simulink model "control_pos_3dof_conMI"  (R2023b)
settings: Solver=ode45  StartTime=0.0  StopTime=tsim  FixedStep=tstep  MaxStep=tstep  RelTol=1e-3
undefined symbols (not defined in the file): a0, a1, MI_Contr1, MI_Contr2, MI_Contr3, MI_motor1, MI_motor2, MI_motor3, robot_params, sigbuilder_block, t_qeq_init, t_tr_init, tau_L
(part 1 of 4)
settings Model: Creator=HP  LastModifiedBy=HP

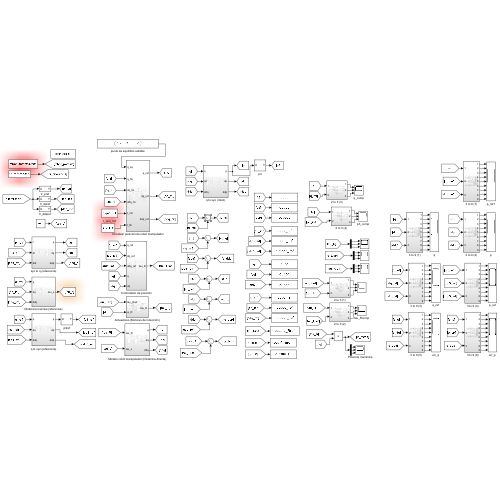
[thumbnail: Simulink's stored preview of the top-level diagram]
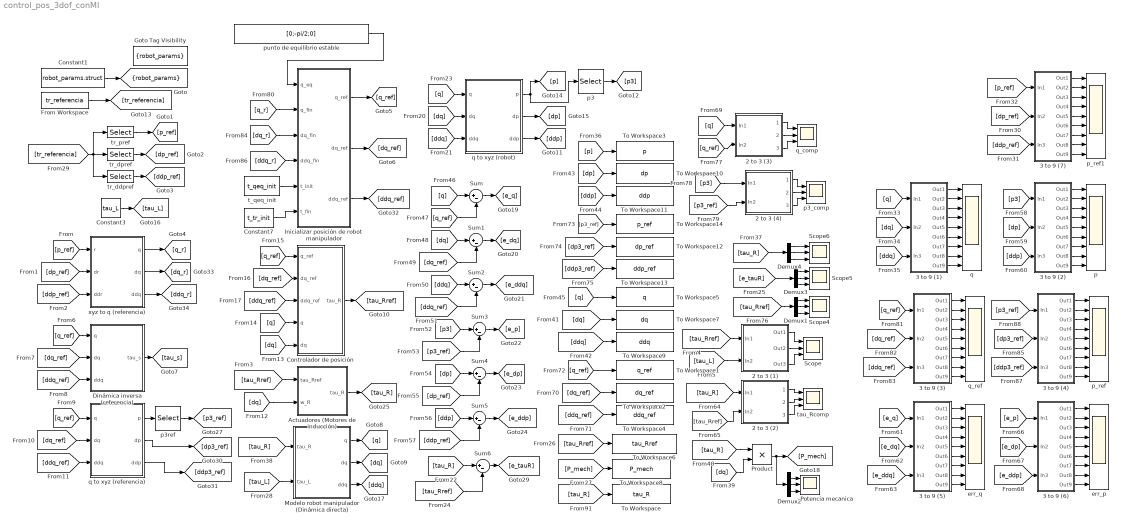
== system control_pos_3dof_conMI ==
  2 to 3 (1) : Subsystem
  2 to 3 (2) : Subsystem
  2 to 3 (3) : Subsystem
  2 to 3 (4) : Subsystem
  3 to 9 (1) : Subsystem
  3 to 9 (2) : Subsystem
  3 to 9 (3) : Subsystem
  3 to 9 (4) : Subsystem
  3 to 9 (5) : Subsystem
  3 to 9 (6) : Subsystem
  3 to 9 (7) : Subsystem
  Actuadores (Motores de inducción) : Subsystem
  Constant1 : Constant  Value=robot_params.struct  OutDataTypeStr=Bus: robot_params_bus
  Constant3 : Constant  Value=tau_L
  Constant7 : Constant  Value=t_tr_init
  Controlador de posición : Subsystem
  Demux{1..4} (4 alike) : Demux  Outputs=3
  Dinámica inversa (referencia) : Subsystem
  From Workspace : FromWorkspace  VariableName=tr_referencia
  Goto Tag Visibility : GotoTagVisibility  GotoTag=robot_params
  Inicializar posición de robot manipulador : Subsystem
  Modelo robot manipulador (Dinámica directa) : Subsystem
  Potencia mecanica : Scope  NumInputPorts=3
  Product : Product
  Scope{,4..6} (4 alike) : Scope  NumInputPorts=3
  Sum{,1..6} (7 alike) : Sum  Inputs=|+-
  To Workspace : ToWorkspace  VariableName=tau_R  SaveFormat=Timeseries  SampleTime=-1
  To Workspace1 : ToWorkspace  VariableName=q_ref  SaveFormat=Timeseries  SampleTime=-1
  To Workspace10 : ToWorkspace  VariableName=dp  SaveFormat=Timeseries  SampleTime=-1
  To Workspace11 : ToWorkspace  VariableName=ddp  SaveFormat=Timeseries  SampleTime=-1
  To Workspace12 : ToWorkspace  VariableName=dp_ref  SaveFormat=Timeseries  SampleTime=-1
  To Workspace13 : ToWorkspace  VariableName=ddp_ref  SaveFormat=Timeseries  SampleTime=-1
  To Workspace14 : ToWorkspace  VariableName=p_ref  SaveFormat=Timeseries  SampleTime=-1
  To Workspace2 : ToWorkspace  VariableName=dq_ref  SaveFormat=Timeseries  SampleTime=-1
  To Workspace3 : ToWorkspace  VariableName=p  SaveFormat=Timeseries  SampleTime=-1
  To Workspace4 : ToWorkspace  VariableName=ddq_ref  SaveFormat=Timeseries  SampleTime=-1
  To Workspace5 : ToWorkspace  VariableName=q  SaveFormat=Timeseries  SampleTime=-1
  To Workspace6 : ToWorkspace  VariableName=tau_Rref  SaveFormat=Timeseries  SampleTime=-1
  To Workspace7 : ToWorkspace  VariableName=dq  SaveFormat=Timeseries  SampleTime=-1
  To Workspace8 : ToWorkspace  VariableName=P_mech  SaveFormat=Timeseries  SampleTime=-1
  To Workspace9 : ToWorkspace  VariableName=ddq  SaveFormat=Timeseries  SampleTime=-1
  err_p : Scope  NumInputPorts=9
  err_q : Scope  NumInputPorts=9
  p : Scope  NumInputPorts=9
  p3 : Selector  NumberOfDimensions=2  InputPortWidth=3  IndexOptions=Index vector (dialog),Index vector (dialog)  Indices=[1:3],3  OutputSizes=1,1
  p3_comp : Scope  NumInputPorts=3
  p3ref : Selector  NumberOfDimensions=2  InputPortWidth=3  IndexOptions=Index vector (dialog),Index vector (dialog)  Indices=[1:3],3  OutputSizes=1,1
  p_ref : Scope  NumInputPorts=9
  p_ref1 : Scope  NumInputPorts=9
  punto de equilibrio estable : Constant  Value=[0;-pi/2;0]
  q : Scope  NumInputPorts=9
  q to xyz (referencia) : Subsystem
  q to xyz (robot) : Subsystem
  q_comp : Scope  NumInputPorts=3
  q_ref : Scope  NumInputPorts=9
  t_qeq_init : Constant  Value=t_qeq_init
  tau_Rcomp : Scope  NumInputPorts=3
  tr_ddpref : Selector  NumberOfDimensions=2  InputPortWidth=3  IndexOptions=Index vector (dialog),Index vector (dialog)  Indices=[7:9],1  OutputSizes=1,1
  tr_dpref : Selector  NumberOfDimensions=2  InputPortWidth=3  IndexOptions=Index vector (dialog),Index vector (dialog)  Indices=[4:6],1  OutputSizes=1,1
  tr_pref : Selector  NumberOfDimensions=2  InputPortWidth=3  IndexOptions=Index vector (dialog),Index vector (dialog)  Indices=[1:3],1  OutputSizes=1,1
  xyz to q (referencia) : Subsystem
  tag scope: robot_params=scoped
  wires:
  From Workspace/1 -> [tr_referencia]
  Constant1/1 -> [robot_params]
  p3/1 -> [p3]
  q to xyz (robot)/2(dp) -> [dp]
  q to xyz (robot)/1(p) -> p3/1, [p]
  [q] -> q to xyz (robot)/1(q)
  [dq] -> q to xyz (robot)/2(dq)
  2 to 3 (1)/2(Out2) -> Scope/2
  [tau_L] -> Modelo robot manipulador (Dinámica directa)/2(tau_L)
  2 to 3 (1)/1(Out1) -> Scope/1
  [tau_R] -> Modelo robot manipulador (Dinámica directa)/1(tau_R)
  [ddq] -> q to xyz (robot)/3(ddq)
  q to xyz (robot)/3(ddp) -> [ddp]
  Constant3/1 -> [tau_L]
  2 to 3 (1)/3(Out3) -> Scope/3
  [tau_R] -> Product/1
  [dq] -> Product/2
  [ddp] -> To Workspace11/1
  Product/1 -> Demux2/1, [P_mech]
  Demux2/3 -> Potencia mecanica/3
  [P_mech] -> To Workspace8/1
  [dq] -> To Workspace7/1
  [q] -> To Workspace5/1
  [tau_Rref] -> To Workspace6/1
  [dp] -> To Workspace10/1
  [p] -> To Workspace3/1
  [ddq] -> To Workspace9/1
  Demux2/2 -> Potencia mecanica/2
  Demux2/1 -> Potencia mecanica/1
  [q] -> Sum/1
  [q_ref] -> Sum/2
  Sum/1 -> [e_q]
  [dq_ref] -> Sum1/2
  Sum1/1 -> [e_dq]
  [dq] -> Sum1/1
  [ddq_ref] -> Sum2/2
  Sum2/1 -> [e_ddq]
  [ddq] -> Sum2/1
  [p3_ref] -> Sum3/2
  Sum4/1 -> [e_dp]
  Sum5/1 -> [e_ddp]
  [ddp_ref] -> Sum5/2
  [dp_ref] -> Sum4/2
  Sum3/1 -> [e_p]
  [p3] -> Sum3/1
  [ddp] -> Sum5/1
  [dp] -> Sum4/1
  p3ref/1 -> [p3_ref]
  [tau_R] -> 2 to 3 (2)/1(In1)
  [tau_Rref] -> 2 to 3 (2)/2(In2)
  2 to 3 (2)/1(1) -> tau_Rcomp/1
  2 to 3 (2)/2(2) -> tau_Rcomp/2
  2 to 3 (2)/3(3) -> tau_Rcomp/3
  [dq_ref] -> To Workspace2/1
  [ddq_ref] -> To Workspace4/1
  [q_ref] -> To Workspace1/1
  [p3_ref] -> To Workspace14/1
  [dp3_ref] -> To Workspace12/1
  [ddp3_ref] -> To Workspace13/1
  [p_ref] -> xyz to q (referencia)/1(r)
  [dp_ref] -> xyz to q (referencia)/2(dr)
  [ddp_ref] -> xyz to q (referencia)/3(ddr)
  [q_ref] -> Dinámica inversa (referencia)/1(q)
  [dq_ref] -> Dinámica inversa (referencia)/2(dq)
  [ddq_ref] -> Dinámica inversa (referencia)/3(ddq)
  Dinámica inversa (referencia)/1(tau_s) -> [tau_s]
  [q_ref] -> q to xyz (referencia)/1(q)
  [dq_ref] -> q to xyz (referencia)/2(dq)
  [ddq_ref] -> q to xyz (referencia)/3(ddq)
  q to xyz (referencia)/1(p) -> p3ref/1
  [tau_Rref] -> 2 to 3 (1)/1(In1)
  [tau_L] -> 2 to 3 (1)/2(In2)
  Modelo robot manipulador (Dinámica directa)/1(q) -> [q]
  Modelo robot manipulador (Dinámica directa)/2(dq) -> [dq]
  Modelo robot manipulador (Dinámica directa)/3(ddq) -> [ddq]
  [q_ref] -> Controlador de posición/1(q_ref)
  [q] -> Controlador de posición/4(q)
  [dq] -> Controlador de posición/5(dq)
  [tr_referencia] -> tr_ddpref/1, tr_pref/1, tr_dpref/1
  tr_pref/1 -> [p_ref]
  tr_dpref/1 -> [dp_ref]
  tr_ddpref/1 -> [ddp_ref]
  [tau_R] -> Sum6/1
  [tau_Rref] -> Sum6/2
  Sum6/1 -> [e_tauR]
  Demux3/3 -> Scope5/3
  Demux3/1 -> Scope5/1
  Demux3/2 -> Scope5/2
  [e_tauR] -> Demux3/1
  Demux1/1 -> Scope4/1
  Demux1/2 -> Scope4/2
  [tau_Rref] -> Demux1/1
  Demux1/3 -> Scope4/3
  [tau_R] -> Demux4/1
  Demux4/1 -> Scope6/1
  Demux4/2 -> Scope6/2
  Demux4/3 -> Scope6/3
  q to xyz (referencia)/2(dp) -> [dp3_ref]
  q to xyz (referencia)/3(ddp) -> [ddp3_ref]
  Controlador de posición/1(tau_R) -> [tau_Rref]
  [dq_ref] -> Controlador de posición/2(dq_ref)
  [ddq_ref] -> Controlador de posición/3(ddq_ref)
  xyz to q (referencia)/2(dq) -> [dq_r]
  xyz to q (referencia)/1(q) -> [q_r]
  xyz to q (referencia)/3(ddq) -> [ddq_r]
  [ddp_ref] -> 3 to 9 (7)/3(In3)
  [dp_ref] -> 3 to 9 (7)/2(In2)
  [p_ref] -> 3 to 9 (7)/1(In1)
  3 to 9 (7)/7(Out7) -> p_ref1/7
  3 to 9 (7)/2(Out2) -> p_ref1/2
  3 to 9 (7)/8(Out8) -> p_ref1/8
  3 to 9 (7)/6(Out6) -> p_ref1/6
  3 to 9 (7)/4(Out4) -> p_ref1/4
  3 to 9 (7)/5(Out5) -> p_ref1/5
  [e_dq] -> 3 to 9 (5)/2(In2)
  2 to 3 (4)/2(2) -> p3_comp/2
  [p3_ref] -> 2 to 3 (4)/2(In2)
  2 to 3 (4)/1(1) -> p3_comp/1
  2 to 3 (3)/3(3) -> q_comp/3
  3 to 9 (5)/6(Out6) -> err_q/6
  3 to 9 (5)/9(Out9) -> err_q/9
  2 to 3 (4)/3(3) -> p3_comp/3
  3 to 9 (6)/3(Out3) -> err_p/3
  3 to 9 (6)/8(Out8) -> err_p/8
  3 to 9 (3)/3(Out3) -> q_ref/3
  3 to 9 (3)/2(Out2) -> q_ref/2
  2 to 3 (3)/1(1) -> q_comp/1
  3 to 9 (5)/5(Out5) -> err_q/5
  3 to 9 (4)/3(Out3) -> p_ref/3
  [ddq_ref] -> 3 to 9 (3)/3(In3)
  3 to 9 (5)/1(Out1) -> err_q/1
  [dq_ref] -> 3 to 9 (3)/2(In2)
  3 to 9 (6)/9(Out9) -> err_p/9
  [e_p] -> 3 to 9 (6)/1(In1)
  3 to 9 (3)/6(Out6) -> q_ref/6
  3 to 9 (4)/2(Out2) -> p_ref/2
  3 to 9 (4)/9(Out9) -> p_ref/9
  3 to 9 (1)/7(Out7) -> q/7
  3 to 9 (3)/8(Out8) -> q_ref/8
  3 to 9 (3)/1(Out1) -> q_ref/1
  3 to 9 (6)/5(Out5) -> err_p/5
  3 to 9 (4)/4(Out4) -> p_ref/4
  3 to 9 (7)/3(Out3) -> p_ref1/3
  3 to 9 (6)/4(Out4) -> err_p/4
  3 to 9 (1)/5(Out5) -> q/5
  3 to 9 (4)/1(Out1) -> p_ref/1
  3 to 9 (3)/9(Out9) -> q_ref/9
  3 to 9 (4)/5(Out5) -> p_ref/5
  [dq] -> 3 to 9 (1)/2(In2)
  3 to 9 (5)/2(Out2) -> err_q/2
  3 to 9 (7)/9(Out9) -> p_ref1/9
  [q_ref] -> 3 to 9 (3)/1(In1)
  [q] -> 2 to 3 (3)/1(In1)
  [e_q] -> 3 to 9 (5)/1(In1)
  3 to 9 (5)/8(Out8) -> err_q/8
  [e_ddp] -> 3 to 9 (6)/3(In3)
  [q_ref] -> 2 to 3 (3)/2(In2)
  3 to 9 (1)/9(Out9) -> q/9
  [p3_ref] -> 3 to 9 (4)/1(In1)
  [e_dp] -> 3 to 9 (6)/2(In2)
  2 to 3 (3)/2(2) -> q_comp/2
  3 to 9 (3)/7(Out7) -> q_ref/7
  3 to 9 (5)/7(Out7) -> err_q/7
  3 to 9 (6)/2(Out2) -> err_p/2
  3 to 9 (2)/7(Out7) -> p/7
  [p3] -> 2 to 3 (4)/1(In1)
  3 to 9 (6)/7(Out7) -> err_p/7
  3 to 9 (4)/8(Out8) -> p_ref/8
  [e_ddq] -> 3 to 9 (5)/3(In3)
  3 to 9 (6)/6(Out6) -> err_p/6
  3 to 9 (4)/7(Out7) -> p_ref/7
  3 to 9 (5)/3(Out3) -> err_q/3
  3 to 9 (3)/5(Out5) -> q_ref/5
  3 to 9 (2)/2(Out2) -> p/2
  3 to 9 (1)/3(Out3) -> q/3
  3 to 9 (2)/4(Out4) -> p/4
  3 to 9 (1)/4(Out4) -> q/4
  [dp3_ref] -> 3 to 9 (4)/2(In2)
  [dp] -> 3 to 9 (2)/2(In2)
  3 to 9 (1)/6(Out6) -> q/6
  3 to 9 (1)/8(Out8) -> q/8
  3 to 9 (1)/1(Out1) -> q/1
  [q] -> 3 to 9 (1)/1(In1)
  3 to 9 (2)/1(Out1) -> p/1
  [p3] -> 3 to 9 (2)/1(In1)
  3 to 9 (2)/6(Out6) -> p/6
  3 to 9 (3)/4(Out4) -> q_ref/4
  3 to 9 (2)/9(Out9) -> p/9
  3 to 9 (2)/3(Out3) -> p/3
  [ddp] -> 3 to 9 (2)/3(In3)
  3 to 9 (2)/8(Out8) -> p/8
  3 to 9 (5)/4(Out4) -> err_q/4
  [ddq] -> 3 to 9 (1)/3(In3)
  3 to 9 (1)/2(Out2) -> q/2
  [ddp3_ref] -> 3 to 9 (4)/3(In3)
  3 to 9 (2)/5(Out5) -> p/5
  3 to 9 (4)/6(Out6) -> p_ref/6
  3 to 9 (6)/1(Out1) -> err_p/1
  3 to 9 (7)/1(Out1) -> p_ref1/1
  [tau_R] -> To Workspace/1
  punto de equilibrio estable/1 -> Inicializar posición de robot manipulador/1(q_eq)
  Inicializar posición de robot manipulador/3(ddq_ref) -> [ddq_ref]
  [ddq_r] -> Inicializar posición de robot manipulador/4(ddq_fin)
  Inicializar posición de robot manipulador/1(q_ref) -> [q_ref]
  Inicializar posición de robot manipulador/2(dq_ref) -> [dq_ref]
  [dq_r] -> Inicializar posición de robot manipulador/3(dq_fin)
  [q_r] -> Inicializar posición de robot manipulador/2(q_fin)
  t_qeq_init/1 -> Inicializar posición de robot manipulador/5(t_init)
  Constant7/1 -> Inicializar posición de robot manipulador/6(t_fin)
  [tau_Rref] -> Actuadores (Motores de inducción)/1(tau_Rref)
  Actuadores (Motores de inducción)/1(tau_R) -> [tau_R]
  [dq] -> Actuadores (Motores de inducción)/2(w_R)

== system control_pos_3dof_conMI/2 to 3 (1) ==
  In1 : Inport
  In2 : Inport  Port=2
  Demux : Demux  Outputs=3
  Demux1 : Demux  Outputs=3
  Mux : Mux  Inputs=2
  Mux1 : Mux  Inputs=2
  Mux2 : Mux  Inputs=2
  Out1 : Outport
  Out2 : Outport  Port=2
  Out3 : Outport  Port=3
  wires:
  Demux/3 -> Mux2/1
  Mux2/1 -> Out3/1
  Mux1/1 -> Out2/1
  Demux/1 -> Mux/1
  Demux1/1 -> Mux/2
  In1/1 -> Demux/1
  Demux/2 -> Mux1/1
  Demux1/2 -> Mux1/2
  Mux/1 -> Out1/1
  Demux1/3 -> Mux2/2
  In2/1 -> Demux1/1

== system control_pos_3dof_conMI/2 to 3 (2) ==
  In1 : Inport
  In2 : Inport  Port=2
  Demux3 : Demux  Outputs=3
  Demux4 : Demux  Outputs=3
  Mux10 : Mux  Inputs=2
  Mux8 : Mux  Inputs=2
  Mux9 : Mux  Inputs=2
  1 : Outport
  2 : Outport  Port=2
  3 : Outport  Port=3
  wires:
  Demux4/3 -> Mux10/2
  Demux3/1 -> Mux8/1
  Demux3/2 -> Mux9/1
  Mux9/1 -> 2/1
  Demux4/2 -> Mux9/2
  Demux4/1 -> Mux8/2
  Demux3/3 -> Mux10/1
  Mux8/1 -> 1/1
  Mux10/1 -> 3/1
  In1/1 -> Demux3/1
  In2/1 -> Demux4/1

== system control_pos_3dof_conMI/2 to 3 (3) ==
  In1 : Inport
  In2 : Inport  Port=2
  Demux3 : Demux  Outputs=3
  Demux4 : Demux  Outputs=3
  Mux10 : Mux  Inputs=2
  Mux8 : Mux  Inputs=2
  Mux9 : Mux  Inputs=2
  1 : Outport
  2 : Outport  Port=2
  3 : Outport  Port=3
  wires:
  Demux4/3 -> Mux10/2
  Demux3/1 -> Mux8/1
  Demux3/2 -> Mux9/1
  Mux9/1 -> 2/1
  Demux4/2 -> Mux9/2
  Demux4/1 -> Mux8/2
  Demux3/3 -> Mux10/1
  Mux8/1 -> 1/1
  Mux10/1 -> 3/1
  In1/1 -> Demux3/1
  In2/1 -> Demux4/1

== system control_pos_3dof_conMI/2 to 3 (4) ==
  In1 : Inport
  In2 : Inport  Port=2
  Demux3 : Demux  Outputs=3
  Demux4 : Demux  Outputs=3
  Mux10 : Mux  Inputs=2
  Mux8 : Mux  Inputs=2
  Mux9 : Mux  Inputs=2
  1 : Outport
  2 : Outport  Port=2
  3 : Outport  Port=3
  wires:
  Demux4/3 -> Mux10/2
  Demux3/1 -> Mux8/1
  Demux3/2 -> Mux9/1
  Mux9/1 -> 2/1
  Demux4/2 -> Mux9/2
  Demux4/1 -> Mux8/2
  Demux3/3 -> Mux10/1
  Mux8/1 -> 1/1
  Mux10/1 -> 3/1
  In1/1 -> Demux3/1
  In2/1 -> Demux4/1

== system control_pos_3dof_conMI/3 to 9 (1) ==
  In1 : Inport
  In2 : Inport  Port=2
  In3 : Inport  Port=3
  Demux2 : Demux  Outputs=3
  Demux3 : Demux  Outputs=3
  Demux4 : Demux  Outputs=3
  Out1 : Outport
  Out2 : Outport  Port=2
  Out3 : Outport  Port=3
  Out4 : Outport  Port=4
  Out5 : Outport  Port=5
  Out6 : Outport  Port=6
  Out7 : Outport  Port=7
  Out8 : Outport  Port=8
  Out9 : Outport  Port=9
  wires:
  In3/1 -> Demux4/1
  Demux4/1 -> Out3/1
  Demux2/1 -> Out1/1
  Demux3/3 -> Out8/1
  Demux3/2 -> Out5/1
  Demux3/1 -> Out2/1
  In1/1 -> Demux2/1
  Demux2/3 -> Out7/1
  Demux4/3 -> Out9/1
  Demux4/2 -> Out6/1
  Demux2/2 -> Out4/1
  In2/1 -> Demux3/1

== system control_pos_3dof_conMI/3 to 9 (2) ==
  In1 : Inport
  In2 : Inport  Port=2
  In3 : Inport  Port=3
  Demux2 : Demux  Outputs=3
  Demux3 : Demux  Outputs=3
  Demux4 : Demux  Outputs=3
  Out1 : Outport
  Out2 : Outport  Port=2
  Out3 : Outport  Port=3
  Out4 : Outport  Port=4
  Out5 : Outport  Port=5
  Out6 : Outport  Port=6
  Out7 : Outport  Port=7
  Out8 : Outport  Port=8
  Out9 : Outport  Port=9
  wires:
  In3/1 -> Demux4/1
  Demux4/1 -> Out3/1
  Demux2/1 -> Out1/1
  Demux3/3 -> Out8/1
  Demux3/2 -> Out5/1
  Demux3/1 -> Out2/1
  In1/1 -> Demux2/1
  Demux2/3 -> Out7/1
  Demux4/3 -> Out9/1
  Demux4/2 -> Out6/1
  Demux2/2 -> Out4/1
  In2/1 -> Demux3/1

== system control_pos_3dof_conMI/3 to 9 (3) ==
  In1 : Inport
  In2 : Inport  Port=2
  In3 : Inport  Port=3
  Demux2 : Demux  Outputs=3
  Demux3 : Demux  Outputs=3
  Demux4 : Demux  Outputs=3
  Out1 : Outport
  Out2 : Outport  Port=2
  Out3 : Outport  Port=3
  Out4 : Outport  Port=4
  Out5 : Outport  Port=5
  Out6 : Outport  Port=6
  Out7 : Outport  Port=7
  Out8 : Outport  Port=8
  Out9 : Outport  Port=9
  wires:
  In3/1 -> Demux4/1
  Demux4/1 -> Out3/1
  Demux2/1 -> Out1/1
  Demux3/3 -> Out8/1
  Demux3/2 -> Out5/1
  Demux3/1 -> Out2/1
  In1/1 -> Demux2/1
  Demux2/3 -> Out7/1
  Demux4/3 -> Out9/1
  Demux4/2 -> Out6/1
  Demux2/2 -> Out4/1
  In2/1 -> Demux3/1

== system control_pos_3dof_conMI/3 to 9 (4) ==
  In1 : Inport
  In2 : Inport  Port=2
  In3 : Inport  Port=3
  Demux2 : Demux  Outputs=3
  Demux3 : Demux  Outputs=3
  Demux4 : Demux  Outputs=3
  Out1 : Outport
  Out2 : Outport  Port=2
  Out3 : Outport  Port=3
  Out4 : Outport  Port=4
  Out5 : Outport  Port=5
  Out6 : Outport  Port=6
  Out7 : Outport  Port=7
  Out8 : Outport  Port=8
  Out9 : Outport  Port=9
  wires:
  In3/1 -> Demux4/1
  Demux4/1 -> Out3/1
  Demux2/1 -> Out1/1
  Demux3/3 -> Out8/1
  Demux3/2 -> Out5/1
  Demux3/1 -> Out2/1
  In1/1 -> Demux2/1
  Demux2/3 -> Out7/1
  Demux4/3 -> Out9/1
  Demux4/2 -> Out6/1
  Demux2/2 -> Out4/1
  In2/1 -> Demux3/1

== system control_pos_3dof_conMI/3 to 9 (5) ==
  In1 : Inport
  In2 : Inport  Port=2
  In3 : Inport  Port=3
  Demux2 : Demux  Outputs=3
  Demux3 : Demux  Outputs=3
  Demux4 : Demux  Outputs=3
  Out1 : Outport
  Out2 : Outport  Port=2
  Out3 : Outport  Port=3
  Out4 : Outport  Port=4
  Out5 : Outport  Port=5
  Out6 : Outport  Port=6
  Out7 : Outport  Port=7
  Out8 : Outport  Port=8
  Out9 : Outport  Port=9
  wires:
  In3/1 -> Demux4/1
  Demux4/1 -> Out3/1
  Demux2/1 -> Out1/1
  Demux3/3 -> Out8/1
  Demux3/2 -> Out5/1
  Demux3/1 -> Out2/1
  In1/1 -> Demux2/1
  Demux2/3 -> Out7/1
  Demux4/3 -> Out9/1
  Demux4/2 -> Out6/1
  Demux2/2 -> Out4/1
  In2/1 -> Demux3/1

== system control_pos_3dof_conMI/3 to 9 (6) ==
  In1 : Inport
  In2 : Inport  Port=2
  In3 : Inport  Port=3
  Demux2 : Demux  Outputs=3
  Demux3 : Demux  Outputs=3
  Demux4 : Demux  Outputs=3
  Out1 : Outport
  Out2 : Outport  Port=2
  Out3 : Outport  Port=3
  Out4 : Outport  Port=4
  Out5 : Outport  Port=5
  Out6 : Outport  Port=6
  Out7 : Outport  Port=7
  Out8 : Outport  Port=8
  Out9 : Outport  Port=9
  wires:
  In3/1 -> Demux4/1
  Demux4/1 -> Out3/1
  Demux2/1 -> Out1/1
  Demux3/3 -> Out8/1
  Demux3/2 -> Out5/1
  Demux3/1 -> Out2/1
  In1/1 -> Demux2/1
  Demux2/3 -> Out7/1
  Demux4/3 -> Out9/1
  Demux4/2 -> Out6/1
  Demux2/2 -> Out4/1
  In2/1 -> Demux3/1

== system control_pos_3dof_conMI/3 to 9 (7) ==
  In1 : Inport
  In2 : Inport  Port=2
  In3 : Inport  Port=3
  Demux2 : Demux  Outputs=3
  Demux3 : Demux  Outputs=3
  Demux4 : Demux  Outputs=3
  Out1 : Outport
  Out2 : Outport  Port=2
  Out3 : Outport  Port=3
  Out4 : Outport  Port=4
  Out5 : Outport  Port=5
  Out6 : Outport  Port=6
  Out7 : Outport  Port=7
  Out8 : Outport  Port=8
  Out9 : Outport  Port=9
  wires:
  In3/1 -> Demux4/1
  Demux4/1 -> Out3/1
  Demux2/1 -> Out1/1
  Demux3/3 -> Out8/1
  Demux3/2 -> Out5/1
  Demux3/1 -> Out2/1
  In1/1 -> Demux2/1
  Demux2/3 -> Out7/1
  Demux4/3 -> Out9/1
  Demux4/2 -> Out6/1
  Demux2/2 -> Out4/1
  In2/1 -> Demux3/1

== system control_pos_3dof_conMI/Actuadores (Motores de inducción) ==
  tau_Rref : Inport
  w_R : Inport  Port=2
  Demux : Demux  Outputs=3
  Demux3 : Demux  Outputs=3
  MI1 + PBC Torque Controller : Subsystem
  MI2 + PBC Torque Controller : Subsystem
  MI3 + PBC Torque Controller : Subsystem
  Mux : Mux  Inputs=3
  tau_R : Outport
  wires:
  Demux3/1 -> MI1 + PBC Torque Controller/2(dq)
  Demux/1 -> MI1 + PBC Torque Controller/1(tau_Rref)
  MI1 + PBC Torque Controller/1(tau_R) -> Mux/1
  Demux3/3 -> MI3 + PBC Torque Controller/2(dq)
  MI2 + PBC Torque Controller/1(tau_R) -> Mux/2
  MI3 + PBC Torque Controller/1(tau_R) -> Mux/3
  Demux3/2 -> MI2 + PBC Torque Controller/2(dq)
  Demux/3 -> MI3 + PBC Torque Controller/1(tau_Rref)
  Demux/2 -> MI2 + PBC Torque Controller/1(tau_Rref)
  tau_Rref/1 -> Demux/1
  w_R/1 -> Demux3/1
  Mux/1 -> tau_R/1

== system control_pos_3dof_conMI/Controlador de posición ==
  q_ref : Inport
  dq_ref : Inport  Port=2
  ddq_ref : Inport  Port=3
  q : Inport  Port=4
  dq : Inport  Port=5
  Constant2 : Constant  Value=a1
  Constant4 : Constant  Value=a0
  Controlador : MATLAB Function  TreatAsAtomicUnit=on
  Controlador no lineal : MATLAB Function  Commented=on  TreatAsAtomicUnit=on
  Modelo dinámico : MATLAB Function  TreatAsAtomicUnit=on
  tau_R : Outport
  wires:
  [dq] -> Modelo dinámico/3(dq)
  [q] -> Modelo dinámico/2(q)
  [robot_params] -> Modelo dinámico/1(robot_params)
  Modelo dinámico/1(robot_din) -> [robot_din]
  dq/1 -> [dq]
  q/1 -> [q]
  ddq_ref/1 -> [ddq_ref]
  dq_ref/1 -> [dq_ref]
  q_ref/1 -> [q_ref]
  [robot_din] -> Controlador/1(robot_din)
  [a0] -> Controlador/2(A0)
  [a1] -> Controlador/3(A1)
  [q_ref] -> Controlador/4(q_ref)
  [dq_ref] -> Controlador/5(dq_ref)
  [ddq_ref] -> Controlador/6(ddq_ref)
  [q] -> Controlador/7(q)
  [dq] -> Controlador/8(dq)
  Controlador/1(tau_R) -> [tau_R]
  [tau_R] -> tau_R/1
  Constant4/1 -> [a0]
  Constant2/1 -> [a1]

== system control_pos_3dof_conMI/Dinámica inversa (referencia) ==
  q : Inport
  dq : Inport  Port=2
  ddq : Inport  Port=3
  Dinamica inversa (referencia) : MATLAB Function  Commented=on  TreatAsAtomicUnit=on
  Dinámica inversa : MATLAB Function  TreatAsAtomicUnit=on
  Modelo dinámico : MATLAB Function  TreatAsAtomicUnit=on
  tau_s : Outport
  wires:
  [dq_ref] -> Modelo dinámico/3(dq)
  [robot_params] -> Modelo dinámico/1(robot_params)
  Modelo dinámico/1(robot_din) -> [robot_din]
  [q_ref] -> Modelo dinámico/2(q)
  q/1 -> [q_ref]
  dq/1 -> [dq_ref]
  Dinámica inversa/1(tau_s) -> [tau_s]
  [robot_din] -> Dinámica inversa/1(robot_din)
  [ddq_ref] -> Dinámica inversa/3(ddq)
  [dq_ref] -> Dinámica inversa/2(dq)
  ddq/1 -> [ddq_ref]
  [tau_s] -> tau_s/1

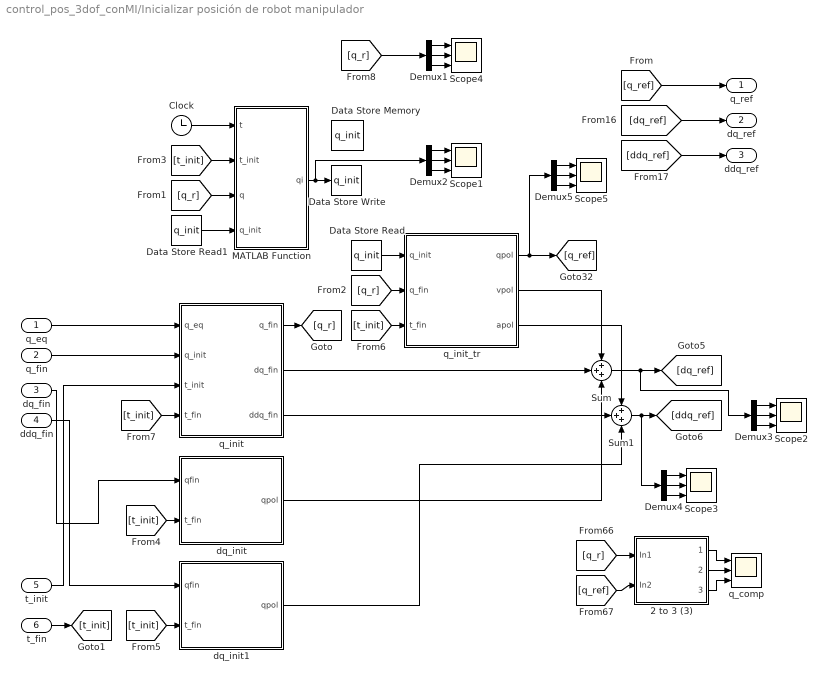
== system control_pos_3dof_conMI/Inicializar posición de robot manipulador ==
  q_eq : Inport
  q_fin : Inport  Port=2
  dq_fin : Inport  Port=3
  ddq_fin : Inport  Port=4
  t_init : Inport  Port=5
  t_fin : Inport  Port=6
  2 to 3 (3) : Subsystem
  Clock : Clock
  Data Store Memory : DataStoreMemory  DataStoreName=q_init  WriteAfterWriteMsg=warning  InitialValue=[0;-pi/2;0]  ShowAdditionalParam=off
  Data Store Read : DataStoreRead  DataStoreName=q_init  IndexOptions=Index vector (dialog)  Indices=1  OutputSizes=1
  Data Store Read1 : DataStoreRead  DataStoreName=q_init  IndexOptions=Index vector (dialog)  Indices=1  OutputSizes=1
  Data Store Write : DataStoreWrite  DataStoreName=q_init  IndexOptions=Index vector (dialog)  Indices=1  OutputSizes=1
  Demux{1..5} (5 alike) : Demux  Outputs=3
  MATLAB Function : MATLAB Function  TreatAsAtomicUnit=on
  Scope{1..5} (5 alike) : Scope  NumInputPorts=3
  Sum : Sum  Inputs=+++
  Sum1 : Sum  Inputs=+++
  dq_init : Subsystem
  dq_init1 : Subsystem
  q_comp : Scope  NumInputPorts=3
  q_init : Subsystem
  q_init_tr : Subsystem
  q_ref : Outport
  dq_ref : Outport  Port=2
  ddq_ref : Outport  Port=3
  wires:
  [ddq_ref] -> ddq_ref/1
  q_fin/1 -> q_init/2(q_init)
  [t_init] -> dq_init/2(t_fin)
  dq_fin/1 -> dq_init/1(qfin)
  [t_init] -> dq_init1/2(t_fin)
  [dq_ref] -> dq_ref/1
  q_eq/1 -> q_init/1(q_eq)
  ddq_fin/1 -> dq_init1/1(qfin)
  [q_ref] -> q_ref/1
  Sum/1 -> Demux3/1, [dq_ref]
  Sum1/1 -> Demux4/1, [ddq_ref]
  q_init_tr/1(qpol) -> Demux5/1, [q_ref]
  [t_init] -> q_init_tr/3(t_fin)
  [t_init] -> MATLAB Function/2(t_init)
  Clock/1 -> MATLAB Function/1(t)
  MATLAB Function/1(qi) -> Demux2/1, Data Store Write/1
  Data Store Read/1 -> q_init_tr/1(q_init)
  Data Store Read1/1 -> MATLAB Function/4(q_init)
  q_init/1(q_fin) -> [q_r]
  [q_r] -> MATLAB Function/3(q)
  [q_r] -> q_init_tr/2(q_fin)
  t_init/1 -> q_init/3(t_init)
  [q_r] -> Demux1/1
  t_fin/1 -> [t_init]
  [t_init] -> q_init/4(t_fin)
  q_init/2(dq_fin) -> Sum/2
  q_init_tr/2(vpol) -> Sum/1
  dq_init/1(qpol) -> Sum/3
  q_init_tr/3(apol) -> Sum1/1
  q_init/3(ddq_fin) -> Sum1/2
  dq_init1/1(qpol) -> Sum1/3
  [q_ref] -> 2 to 3 (3)/2(In2)
  2 to 3 (3)/2(2) -> q_comp/2
  [q_r] -> 2 to 3 (3)/1(In1)
  2 to 3 (3)/3(3) -> q_comp/3
  2 to 3 (3)/1(1) -> q_comp/1
  Demux1/3 -> Scope4/3
  Demux1/1 -> Scope4/1
  Demux1/2 -> Scope4/2
  Demux2/3 -> Scope1/3
  Demux2/1 -> Scope1/1
  Demux2/2 -> Scope1/2
  Demux3/3 -> Scope2/3
  Demux3/1 -> Scope2/1
  Demux3/2 -> Scope2/2
  Demux4/3 -> Scope3/3
  Demux4/1 -> Scope3/1
  Demux4/2 -> Scope3/2
  Demux5/3 -> Scope5/3
  Demux5/1 -> Scope5/1
  Demux5/2 -> Scope5/2

== system control_pos_3dof_conMI/Modelo robot manipulador (Dinámica directa) ==
  tau_R : Inport
  tau_L : Inport  Port=2
  Dinámica directa : MATLAB Function  TreatAsAtomicUnit=on
  Dinámica directa(1) : MATLAB Function  Commented=on  TreatAsAtomicUnit=on
  Modelo dinámico : MATLAB Function  TreatAsAtomicUnit=on
  Scope : Scope
  int_ddq : Integrator  InitialCondition=[0;0;0]
  int_dq : Integrator  InitialCondition=[0;-1.5708;0]
  q : Outport
  dq : Outport  Port=2
  ddq : Outport  Port=3
  wires:
  [robot_params] -> Modelo dinámico/1(robot_params)
  [dq] -> Modelo dinámico/3(dq)
  Modelo dinámico/1(robot_din) -> [robot_din]
  [q] -> Modelo dinámico/2(q)
  [tau_L] -> Dinámica directa/4(tau_L)
  int_ddq/1 -> [dq], int_dq/1
  [robot_din] -> Dinámica directa/1(robot_din)
  [dq] -> Dinámica directa/2(dq)
  int_dq/1 -> [q]
  [tau_R] -> Dinámica directa/3(tau_R)
  [q] -> q/1
  [dq] -> dq/1
  [ddq] -> ddq/1
  tau_R/1 -> [tau_R]
  tau_L/1 -> [tau_L]
  Dinámica directa/1(ddq) -> Scope/1, [ddq], int_ddq/1

== system control_pos_3dof_conMI/q to xyz (referencia) ==
  q : Inport
  dq : Inport  Port=2
  ddq : Inport  Port=3
  Cinemática directa : MATLAB Function  TreatAsAtomicUnit=on
  Jacobiano : MATLAB Function  TreatAsAtomicUnit=on
  ddq to ddp : MATLAB Function  TreatAsAtomicUnit=on
  derivada Jacobiano : MATLAB Function  TreatAsAtomicUnit=on
  dq to dp : MATLAB Function  TreatAsAtomicUnit=on
  q to xyz (referencia) : MATLAB Function  Commented=on  TreatAsAtomicUnit=on
  p : Outport
  dp : Outport  Port=2
  ddp : Outport  Port=3
  wires:
  q/1 -> [q_ref]
  ddq/1 -> [ddq_ref]
  dq/1 -> [dq_ref]
  [dq_ref] -> derivada Jacobiano/3(dq)
  derivada Jacobiano/1(dJP) -> [dJPref]
  [robot_params] -> derivada Jacobiano/1(robot_params)
  [q_ref] -> derivada Jacobiano/2(q)
  [q_ref] -> Cinemática directa/2(q)
  [robot_params] -> Cinemática directa/1(robot_params)
  [robot_params] -> Jacobiano/1(robot_params)
  [q_ref] -> Jacobiano/2(q)
  Jacobiano/1(JP) -> [JP]
  dq to dp/1(dp) -> dp/1
  [dq_ref] -> dq to dp/2(dq)
  [dJPref] -> ddq to ddp/1(dJP)
  [JP] -> dq to dp/1(JP)
  ddq to ddp/1(ddp) -> ddp/1
  [ddq_ref] -> ddq to ddp/2(ddq)
  Cinemática directa/1(p) -> p/1

== system control_pos_3dof_conMI/q to xyz (robot) ==
  q : Inport
  dq : Inport  Port=2
  ddq : Inport  Port=3
  Cinemática directa : MATLAB Function  TreatAsAtomicUnit=on
  Jacobiano : MATLAB Function  TreatAsAtomicUnit=on
  ddq to ddp : MATLAB Function  TreatAsAtomicUnit=on
  derivada Jacobiano : MATLAB Function  TreatAsAtomicUnit=on
  dq to dp : MATLAB Function  TreatAsAtomicUnit=on
  q to xyz (referencia) : MATLAB Function  Commented=on  TreatAsAtomicUnit=on
  p : Outport
  dp : Outport  Port=2
  ddp : Outport  Port=3
  wires:
  q/1 -> [q]
  ddq/1 -> [ddq]
  dq/1 -> [dq]
  [dq] -> derivada Jacobiano/3(dq)
  derivada Jacobiano/1(dJP) -> [dJPref]
  [robot_params] -> derivada Jacobiano/1(robot_params)
  [q] -> derivada Jacobiano/2(q)
  [q] -> Cinemática directa/2(q)
  [robot_params] -> Cinemática directa/1(robot_params)
  [robot_params] -> Jacobiano/1(robot_params)
  [q] -> Jacobiano/2(q)
  Jacobiano/1(JP) -> [JP]
  dq to dp/1(dp) -> dp/1
  [dq] -> dq to dp/2(dq)
  [dJPref] -> ddq to ddp/1(dJP)
  [JP] -> dq to dp/1(JP)
  ddq to ddp/1(ddp) -> ddp/1
  [ddq] -> ddq to ddp/2(ddq)
  Cinemática directa/1(p) -> p/1

== system control_pos_3dof_conMI/xyz to q (referencia) ==
  r : Inport
  dr : Inport  Port=2
  ddr : Inport  Port=3
  Cinemática inversa : MATLAB Function  TreatAsAtomicUnit=on
  Jacobiano inverso : MATLAB Function  TreatAsAtomicUnit=on
  ddr to ddq : MATLAB Function  TreatAsAtomicUnit=on
  derivada Jacobiano : MATLAB Function  TreatAsAtomicUnit=on
  dr to dq : MATLAB Function  TreatAsAtomicUnit=on
  xyz to q (referencia) : MATLAB Function  Commented=on  TreatAsAtomicUnit=on
  q : Outport
  dq : Outport  Port=2
  ddq : Outport  Port=3
  wires:
  r/1 -> [r]
  dr/1 -> [dr]
  ddr/1 -> [ddr]
  [robot_params] -> Cinemática inversa/1(robot_params)
  ddr to ddq/1(ddq) -> [ddq_ref]
  [robot_params] -> derivada Jacobiano/1(robot_params)
  [robot_params] -> Jacobiano inverso/1(robot_params)
  dr to dq/1(dq) -> [dq_ref]
  derivada Jacobiano/1(dJP) -> [dJPref]
  [r] -> Cinemática inversa/2(r)
  [dr] -> dr to dq/2(dr)
  [JPinvref] -> dr to dq/1(JPinv)
  [q_ref] -> derivada Jacobiano/2(q)
  [dq_ref] -> derivada Jacobiano/3(dq)
  Jacobiano inverso/1(JPinv) -> [JPinvref]
  [ddr] -> ddr to ddq/4(ddr)
  [JPinvref] -> ddr to ddq/1(JPinv)
  [dq_ref] -> ddr to ddq/3(dq)
  [dJPref] -> ddr to ddq/2(dJP)
  [q_ref] -> Jacobiano inverso/2(q)
  Cinemática inversa/1(q) -> [q_ref]
  [q_ref] -> q/1
  [dq_ref] -> dq/1
  [ddq_ref] -> ddq/1

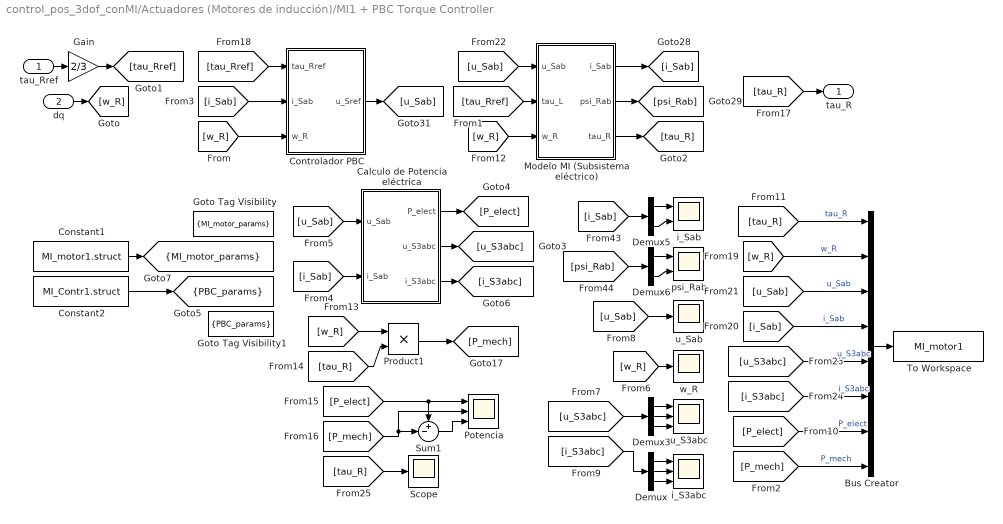
== system control_pos_3dof_conMI/Actuadores (Motores de inducción)/MI1 + PBC Torque Controller ==
  tau_Rref : Inport
  dq : Inport  Port=2
  Bus Creator : BusCreator  Inputs=8
  Calculo de Potencia eléctrica : Subsystem
  Constant1 : Constant  Value=MI_motor1.struct  OutDataTypeStr=Bus: MI_bus
  Constant2 : Constant  Value=MI_Contr1.struct  OutDataTypeStr=Bus: PBC_bus
  Controlador PBC : Subsystem
  Demux : Demux  Outputs=3
  Demux3 : Demux  Outputs=3
  Demux5 : Demux  Outputs=2
  Demux6 : Demux  Outputs=2
  Gain : Gain  Gain=2/3
  Goto Tag Visibility : GotoTagVisibility  GotoTag=MI_motor_params
  Goto Tag Visibility1 : GotoTagVisibility  GotoTag=PBC_params
  Modelo MI (Subsistema eléctrico) : Subsystem
  Potencia : Scope  NumInputPorts=3
  Product1 : Product
  Scope : Scope
  Sum1 : Sum  Inputs=+-|
  To Workspace : ToWorkspace  VariableName=MI_motor1  SaveFormat=Timeseries  SampleTime=-1
  i_S3abc : Scope  NumInputPorts=3
  i_Sab : Scope  NumInputPorts=2
  psi_Rab : Scope  NumInputPorts=2
  u_S3abc : Scope  NumInputPorts=3
  u_Sab : Scope
  w_R : Scope
  tau_R : Outport
  tag scope: MI_motor_params=scoped, PBC_params=scoped
  wires:
  Modelo MI (Subsistema eléctrico)/2(psi_Rab) -> [psi_Rab]
  [u_Sab] -> Modelo MI (Subsistema eléctrico)/1(u_Sab)
  [i_Sab] -> Controlador PBC/2(i_Sab)
  Controlador PBC/1(u_Sref) -> [u_Sab]
  [w_R] -> Controlador PBC/3(w_R)
  [tau_Rref] -> Modelo MI (Subsistema eléctrico)/2(tau_L)
  Calculo de Potencia eléctrica/2(u_S3abc) -> [u_S3abc]
  Calculo de Potencia eléctrica/1(P_elect) -> [P_elect]
  Demux5/1 -> i_Sab/1
  [w_R] -> w_R/1
  [u_Sab] -> Calculo de Potencia eléctrica/1(u_Sab)
  [psi_Rab] -> Demux6/1
  [u_Sab] -> u_Sab/1
  Demux6/1 -> psi_Rab/1
  Calculo de Potencia eléctrica/3(i_S3abc) -> [i_S3abc]
  Demux6/2 -> psi_Rab/2
  Demux5/2 -> i_Sab/2
  [i_Sab] -> Calculo de Potencia eléctrica/2(i_Sab)
  [i_Sab] -> Demux5/1
  Demux/2 -> i_S3abc/2
  Demux3/1 -> u_S3abc/1
  Demux3/3 -> u_S3abc/3
  [i_S3abc] -> Demux/1
  Demux/1 -> i_S3abc/1
  Demux/3 -> i_S3abc/3
  [u_S3abc] -> Demux3/1
  Demux3/2 -> u_S3abc/2
  Modelo MI (Subsistema eléctrico)/1(i_Sab) -> [i_Sab]
  Modelo MI (Subsistema eléctrico)/3(tau_R) -> [tau_R]
  Product1/1 -> [P_mech]
  [w_R] -> Product1/1
  [tau_R] -> Product1/2
  [tau_R] -> Bus Creator/1  "tau_R"
  Sum1/1 -> Potencia/3
  [P_elect] -> Potencia/1, Sum1/1
  [P_mech] -> Potencia/2, Sum1/2
  [tau_R] -> tau_R/1
  dq/1 -> [w_R]
  [tau_Rref] -> Controlador PBC/1(tau_Rref)
  [w_R] -> Modelo MI (Subsistema eléctrico)/3(w_R)
  Bus Creator/1 -> To Workspace/1
  Constant1/1 -> [MI_motor_params]
  [tau_R] -> Scope/1
  Constant2/1 -> [PBC_params]
  [w_R] -> Bus Creator/2  "w_R"
  [u_Sab] -> Bus Creator/3  "u_Sab"
  [i_Sab] -> Bus Creator/4  "i_Sab"
  [u_S3abc] -> Bus Creator/5  "u_S3abc"
  [i_S3abc] -> Bus Creator/6  "i_S3abc"
  [P_elect] -> Bus Creator/7  "P_elect"
  [P_mech] -> Bus Creator/8  "P_mech"
  tau_Rref/1 -> Gain/1
  Gain/1 -> [tau_Rref]

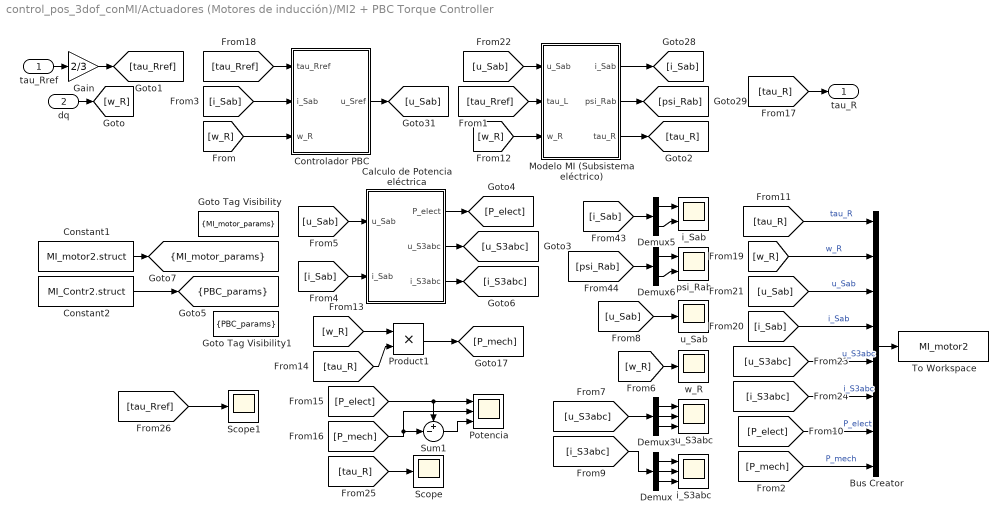
== system control_pos_3dof_conMI/Actuadores (Motores de inducción)/MI2 + PBC Torque Controller ==
  tau_Rref : Inport
  dq : Inport  Port=2
  Bus Creator : BusCreator  Inputs=8
  Calculo de Potencia eléctrica : Subsystem
  Constant1 : Constant  Value=MI_motor2.struct  OutDataTypeStr=Bus: MI_bus
  Constant2 : Constant  Value=MI_Contr2.struct  OutDataTypeStr=Bus: PBC_bus
  Controlador PBC : Subsystem
  Demux : Demux  Outputs=3
  Demux3 : Demux  Outputs=3
  Demux5 : Demux  Outputs=2
  Demux6 : Demux  Outputs=2
  Gain : Gain  Gain=2/3
  Goto Tag Visibility : GotoTagVisibility  GotoTag=MI_motor_params
  Goto Tag Visibility1 : GotoTagVisibility  GotoTag=PBC_params
  Modelo MI (Subsistema eléctrico) : Subsystem
  Potencia : Scope  NumInputPorts=3
  Product1 : Product
  Scope : Scope
  Scope1 : Scope
  Sum1 : Sum  Inputs=+-|
  To Workspace : ToWorkspace  VariableName=MI_motor2  SaveFormat=Timeseries  SampleTime=-1
  i_S3abc : Scope  NumInputPorts=3
  i_Sab : Scope  NumInputPorts=2
  psi_Rab : Scope  NumInputPorts=2
  u_S3abc : Scope  NumInputPorts=3
  u_Sab : Scope
  w_R : Scope
  tau_R : Outport
  tag scope: MI_motor_params=scoped, PBC_params=scoped
  wires:
  Modelo MI (Subsistema eléctrico)/2(psi_Rab) -> [psi_Rab]
  [u_Sab] -> Modelo MI (Subsistema eléctrico)/1(u_Sab)
  [i_Sab] -> Controlador PBC/2(i_Sab)
  Controlador PBC/1(u_Sref) -> [u_Sab]
  [w_R] -> Controlador PBC/3(w_R)
  [tau_Rref] -> Modelo MI (Subsistema eléctrico)/2(tau_L)
  Calculo de Potencia eléctrica/2(u_S3abc) -> [u_S3abc]
  Calculo de Potencia eléctrica/1(P_elect) -> [P_elect]
  Demux5/1 -> i_Sab/1
  [w_R] -> w_R/1
  [u_Sab] -> Calculo de Potencia eléctrica/1(u_Sab)
  [psi_Rab] -> Demux6/1
  [u_Sab] -> u_Sab/1
  Demux6/1 -> psi_Rab/1
  Calculo de Potencia eléctrica/3(i_S3abc) -> [i_S3abc]
  Demux6/2 -> psi_Rab/2
  Demux5/2 -> i_Sab/2
  [i_Sab] -> Calculo de Potencia eléctrica/2(i_Sab)
  [i_Sab] -> Demux5/1
  Demux/2 -> i_S3abc/2
  Demux3/1 -> u_S3abc/1
  Demux3/3 -> u_S3abc/3
  [i_S3abc] -> Demux/1
  Demux/1 -> i_S3abc/1
  Demux/3 -> i_S3abc/3
  [u_S3abc] -> Demux3/1
  Demux3/2 -> u_S3abc/2
  Modelo MI (Subsistema eléctrico)/1(i_Sab) -> [i_Sab]
  Modelo MI (Subsistema eléctrico)/3(tau_R) -> [tau_R]
  Product1/1 -> [P_mech]
  [w_R] -> Product1/1
  [tau_R] -> Product1/2
  [tau_R] -> Bus Creator/1  "tau_R"
  Sum1/1 -> Potencia/3
  [P_elect] -> Potencia/1, Sum1/1
  [P_mech] -> Potencia/2, Sum1/2
  [tau_R] -> tau_R/1
  dq/1 -> [w_R]
  [tau_Rref] -> Controlador PBC/1(tau_Rref)
  [w_R] -> Modelo MI (Subsistema eléctrico)/3(w_R)
  Bus Creator/1 -> To Workspace/1
  Constant1/1 -> [MI_motor_params]
  [tau_R] -> Scope/1
  Constant2/1 -> [PBC_params]
  [w_R] -> Bus Creator/2  "w_R"
  [u_Sab] -> Bus Creator/3  "u_Sab"
  [i_Sab] -> Bus Creator/4  "i_Sab"
  [u_S3abc] -> Bus Creator/5  "u_S3abc"
  [i_S3abc] -> Bus Creator/6  "i_S3abc"
  [P_elect] -> Bus Creator/7  "P_elect"
  [P_mech] -> Bus Creator/8  "P_mech"
  [tau_Rref] -> Scope1/1
  Gain/1 -> [tau_Rref]
  tau_Rref/1 -> Gain/1

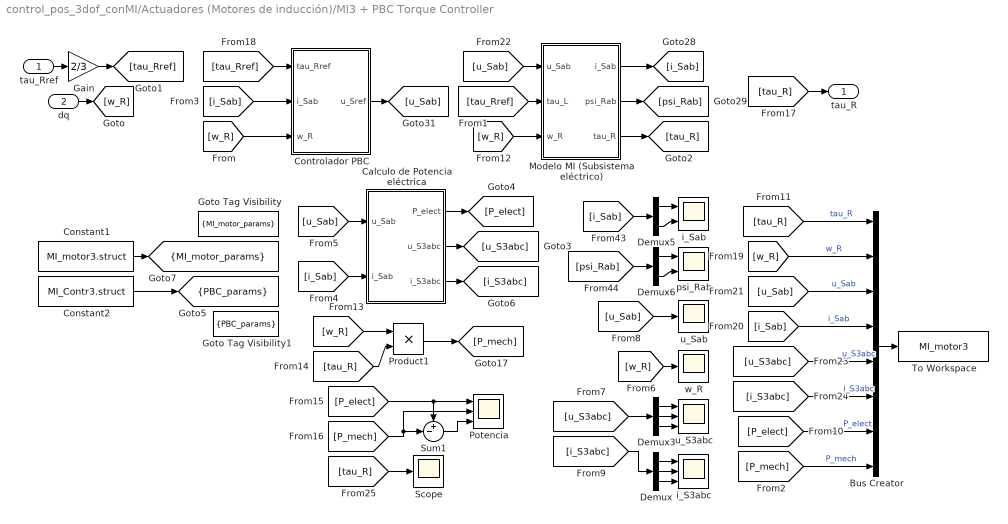
== system control_pos_3dof_conMI/Actuadores (Motores de inducción)/MI3 + PBC Torque Controller ==
  tau_Rref : Inport
  dq : Inport  Port=2
  Bus Creator : BusCreator  Inputs=8
  Calculo de Potencia eléctrica : Subsystem
  Constant1 : Constant  Value=MI_motor3.struct  OutDataTypeStr=Bus: MI_bus
  Constant2 : Constant  Value=MI_Contr3.struct  OutDataTypeStr=Bus: PBC_bus
  Controlador PBC : Subsystem
  Demux : Demux  Outputs=3
  Demux3 : Demux  Outputs=3
  Demux5 : Demux  Outputs=2
  Demux6 : Demux  Outputs=2
  Gain : Gain  Gain=2/3
  Goto Tag Visibility : GotoTagVisibility  GotoTag=MI_motor_params
  Goto Tag Visibility1 : GotoTagVisibility  GotoTag=PBC_params
  Modelo MI (Subsistema eléctrico) : Subsystem
  Potencia : Scope  NumInputPorts=3
  Product1 : Product
  Scope : Scope
  Sum1 : Sum  Inputs=+-|
  To Workspace : ToWorkspace  VariableName=MI_motor3  SaveFormat=Timeseries  SampleTime=-1
  i_S3abc : Scope  NumInputPorts=3
  i_Sab : Scope  NumInputPorts=2
  psi_Rab : Scope  NumInputPorts=2
  u_S3abc : Scope  NumInputPorts=3
  u_Sab : Scope
  w_R : Scope
  tau_R : Outport
  tag scope: MI_motor_params=scoped, PBC_params=scoped
  wires:
  Modelo MI (Subsistema eléctrico)/2(psi_Rab) -> [psi_Rab]
  [u_Sab] -> Modelo MI (Subsistema eléctrico)/1(u_Sab)
  [i_Sab] -> Controlador PBC/2(i_Sab)
  Controlador PBC/1(u_Sref) -> [u_Sab]
  [w_R] -> Controlador PBC/3(w_R)
  [tau_Rref] -> Modelo MI (Subsistema eléctrico)/2(tau_L)
  Calculo de Potencia eléctrica/2(u_S3abc) -> [u_S3abc]
  Calculo de Potencia eléctrica/1(P_elect) -> [P_elect]
  Demux5/1 -> i_Sab/1
  [w_R] -> w_R/1
  [u_Sab] -> Calculo de Potencia eléctrica/1(u_Sab)
  [psi_Rab] -> Demux6/1
  [u_Sab] -> u_Sab/1
  Demux6/1 -> psi_Rab/1
  Calculo de Potencia eléctrica/3(i_S3abc) -> [i_S3abc]
  Demux6/2 -> psi_Rab/2
  Demux5/2 -> i_Sab/2
  [i_Sab] -> Calculo de Potencia eléctrica/2(i_Sab)
  [i_Sab] -> Demux5/1
  Demux/2 -> i_S3abc/2
  Demux3/1 -> u_S3abc/1
  Demux3/3 -> u_S3abc/3
  [i_S3abc] -> Demux/1
  Demux/1 -> i_S3abc/1
  Demux/3 -> i_S3abc/3
  [u_S3abc] -> Demux3/1
  Demux3/2 -> u_S3abc/2
  Modelo MI (Subsistema eléctrico)/1(i_Sab) -> [i_Sab]
  Modelo MI (Subsistema eléctrico)/3(tau_R) -> [tau_R]
  Product1/1 -> [P_mech]
  [w_R] -> Product1/1
  [tau_R] -> Product1/2
  [tau_R] -> Bus Creator/1  "tau_R"
  Sum1/1 -> Potencia/3
  [P_elect] -> Potencia/1, Sum1/1
  [P_mech] -> Potencia/2, Sum1/2
  [tau_R] -> tau_R/1
  dq/1 -> [w_R]
  [tau_Rref] -> Controlador PBC/1(tau_Rref)
  [w_R] -> Modelo MI (Subsistema eléctrico)/3(w_R)
  Bus Creator/1 -> To Workspace/1
  Constant1/1 -> [MI_motor_params]
  [tau_R] -> Scope/1
  Constant2/1 -> [PBC_params]
  [w_R] -> Bus Creator/2  "w_R"
  [u_Sab] -> Bus Creator/3  "u_Sab"
  [i_Sab] -> Bus Creator/4  "i_Sab"
  [u_S3abc] -> Bus Creator/5  "u_S3abc"
  [i_S3abc] -> Bus Creator/6  "i_S3abc"
  [P_elect] -> Bus Creator/7  "P_elect"
  [P_mech] -> Bus Creator/8  "P_mech"
  Gain/1 -> [tau_Rref]
  tau_Rref/1 -> Gain/1

== system control_pos_3dof_conMI/Inicializar posición de robot manipulador/2 to 3 (3) ==
  In1 : Inport
  In2 : Inport  Port=2
  Demux3 : Demux  Outputs=3
  Demux4 : Demux  Outputs=3
  Mux10 : Mux  Inputs=2
  Mux8 : Mux  Inputs=2
  Mux9 : Mux  Inputs=2
  1 : Outport
  2 : Outport  Port=2
  3 : Outport  Port=3
  wires:
  Demux4/3 -> Mux10/2
  Demux3/1 -> Mux8/1
  Demux3/2 -> Mux9/1
  Mux9/1 -> 2/1
  Demux4/2 -> Mux9/2
  Demux4/1 -> Mux8/2
  Demux3/3 -> Mux10/1
  Mux8/1 -> 1/1
  Mux10/1 -> 3/1
  In1/1 -> Demux3/1
  In2/1 -> Demux4/1

== system control_pos_3dof_conMI/Inicializar posición de robot manipulador/dq_init ==
  qfin : Inport
  t_fin : Inport  Port=2
  Demux : Demux  Outputs=3
  Mux : Mux  Inputs=3
  q1 : Subsystem
  q2 : Subsystem
  q3 : Subsystem
  qpol : Outport
  wires:
  qfin/1 -> Demux/1
  t_fin/1 -> [t_fin]
  [t_fin] -> q1/2(t_fin)
  [t_fin] -> q2/2(t_fin)
  [t_fin] -> q3/2(t_fin)
  Mux/1 -> qpol/1
  Demux/1 -> q1/1(q_fin)
  Demux/2 -> q2/1(q_fin)
  Demux/3 -> q3/1(q_fin)
  q1/1(qpol) -> Mux/1
  q2/1(qpol) -> Mux/2
  q3/1(qpol) -> Mux/3

== system control_pos_3dof_conMI/Inicializar posición de robot manipulador/dq_init1 ==
  qfin : Inport
  t_fin : Inport  Port=2
  Demux : Demux  Outputs=3
  Mux : Mux  Inputs=3
  q1 : Subsystem
  q2 : Subsystem
  q3 : Subsystem
  qpol : Outport
  wires:
  qfin/1 -> Demux/1
  t_fin/1 -> [t_fin]
  [t_fin] -> q1/2(t_fin)
  [t_fin] -> q2/2(t_fin)
  [t_fin] -> q3/2(t_fin)
  Mux/1 -> qpol/1
  Demux/1 -> q1/1(q_fin)
  Demux/2 -> q2/1(q_fin)
  Demux/3 -> q3/1(q_fin)
  q1/1(qpol) -> Mux/1
  q2/1(qpol) -> Mux/2
  q3/1(qpol) -> Mux/3

== system control_pos_3dof_conMI/Inicializar posición de robot manipulador/q_init ==
  q_eq : Inport
  q_init : Inport  Port=2
  t_init : Inport  Port=3
  t_fin : Inport  Port=4
  Clock : Clock
  Demux : Demux  Outputs=3
  Demux1 : Demux  Outputs=3
  Mux : Mux  Inputs=3
  Mux1 : Mux  Inputs=3
  Mux2 : Mux  Inputs=3
  init_q1 : Subsystem
  init_q2 : Subsystem
  init_q3 : Subsystem
  q_fin : Outport
  dq_fin : Outport  Port=2
  ddq_fin : Outport  Port=3
  wires:
  t_fin/1 -> [tfin]
  [tfin] -> init_q1/5(t_fin)
  [tfin] -> init_q2/5(t_fin)
  [tfin] -> init_q3/5(t_fin)
  q_eq/1 -> Demux/1
  q_init/1 -> Demux1/1
  Demux/1 -> init_q1/2(q_eq)
  Demux/2 -> init_q2/2(q_eq)
  [t] -> init_q1/1(t)
  [t] -> init_q2/1(t)
  [t] -> init_q3/1(t)
  Demux/3 -> init_q3/2(q_eq)
  t_init/1 -> [t_init]
  [t_init] -> init_q1/4(t_init)
  [t_init] -> init_q2/4(t_init)
  [t_init] -> init_q3/4(t_init)
  Clock/1 -> [t]
  Demux1/1 -> init_q1/3(q_init)
  Demux1/2 -> init_q2/3(q_init)
  Demux1/3 -> init_q3/3(q_init)
  init_q1/1(qpol) -> Mux/1
  init_q2/1(qpol) -> Mux/2
  init_q3/1(qpol) -> Mux/3
  init_q1/2(vpol) -> Mux1/1
  init_q2/2(vpol) -> Mux1/2
  init_q3/2(vpol) -> Mux1/3
  init_q3/3(apol) -> Mux2/3
  init_q2/3(apol) -> Mux2/2
  init_q1/3(apol) -> Mux2/1
  Mux/1 -> q_fin/1
  Mux1/1 -> dq_fin/1
  Mux2/1 -> ddq_fin/1

== system control_pos_3dof_conMI/Inicializar posición de robot manipulador/q_init_tr ==
  q_init : Inport
  q_fin : Inport  Port=2
  t_fin : Inport  Port=3
  Demux : Demux  Outputs=3
  Demux1 : Demux  Outputs=3
  Mux : Mux  Inputs=3
  Mux1 : Mux  Inputs=3
  Mux2 : Mux  Inputs=3
  q1 : Subsystem
  q2 : Subsystem
  q3 : Subsystem
  qpol : Outport
  vpol : Outport  Port=2
  apol : Outport  Port=3
  wires:
  q_fin/1 -> Demux/1
  t_fin/1 -> [t_fin]
  [t_fin] -> q1/3(t_fin)
  [t_fin] -> q2/3(t_fin)
  [t_fin] -> q3/3(t_fin)
  Mux/1 -> qpol/1
  Demux/1 -> q1/2(q_fin)
  Demux/2 -> q2/2(q_fin)
  Demux/3 -> q3/2(q_fin)
  q1/1(qpol) -> Mux/1
  q_init/1 -> Demux1/1
  Demux1/1 -> q1/1(q_init)
  Demux1/2 -> q2/1(q_init)
  Demux1/3 -> q3/1(q_init)
  q2/1(qpol) -> Mux/2
  q3/1(qpol) -> Mux/3
  Mux1/1 -> vpol/1
  Mux2/1 -> apol/1
  q1/2(vpol) -> Mux1/1
  q2/2(vpol) -> Mux1/2
  q3/2(vpol) -> Mux1/3
  q1/3(apol) -> Mux2/1
  q2/3(apol) -> Mux2/2
  q3/3(apol) -> Mux2/3

== system control_pos_3dof_conMI/Actuadores (Motores de inducción)/MI1 + PBC Torque Controller/Calculo de Potencia eléctrica ==
  u_Sab : Inport
  i_Sab : Inport  Port=2
  Blondel-Park-i_Sab : MATLAB Function  TreatAsAtomicUnit=on
  Blondel-Park-u_Sab : MATLAB Function  TreatAsAtomicUnit=on
  Demux1 : Demux  Outputs=2
  Demux2 : Demux  Outputs=2
  Demux4 : Demux  Outputs=3
  Mux : Mux  Inputs=3
  Mux1 : Mux  Inputs=3
  Product1 : Product
  Sum1 : Sum  Inputs=|+++
  P_elect : Outport
  u_S3abc : Outport  Port=2
  i_S3abc : Outport  Port=3
  wires:
  Blondel-Park-u_Sab/2(U2) -> Mux1/2
  Blondel-Park-i_Sab/2(U2) -> Mux/2
  Blondel-Park-i_Sab/1(U1) -> Mux/1
  Blondel-Park-u_Sab/3(U3) -> Mux1/3
  Blondel-Park-i_Sab/3(U3) -> Mux/3
  Sum1/1 -> P_elect/1
  Demux2/2 -> Blondel-Park-u_Sab/2(BPU2)
  Demux2/1 -> Blondel-Park-u_Sab/1(BPU1)
  Demux1/2 -> Blondel-Park-i_Sab/2(BPU2)
  Demux4/1 -> Sum1/1
  [i_S3abc] -> Product1/2
  i_Sab/1 -> Demux2/1
  Blondel-Park-u_Sab/1(U1) -> Mux1/1
  Demux1/1 -> Blondel-Park-i_Sab/1(BPU1)
  Demux4/3 -> Sum1/3
  [u_S3abc] -> Product1/1
  Demux4/2 -> Sum1/2
  Product1/1 -> Demux4/1
  u_Sab/1 -> Demux1/1
  [u_S3abc] -> u_S3abc/1
  [i_S3abc] -> i_S3abc/1
  Mux/1 -> [u_S3abc]
  Mux1/1 -> [i_S3abc]

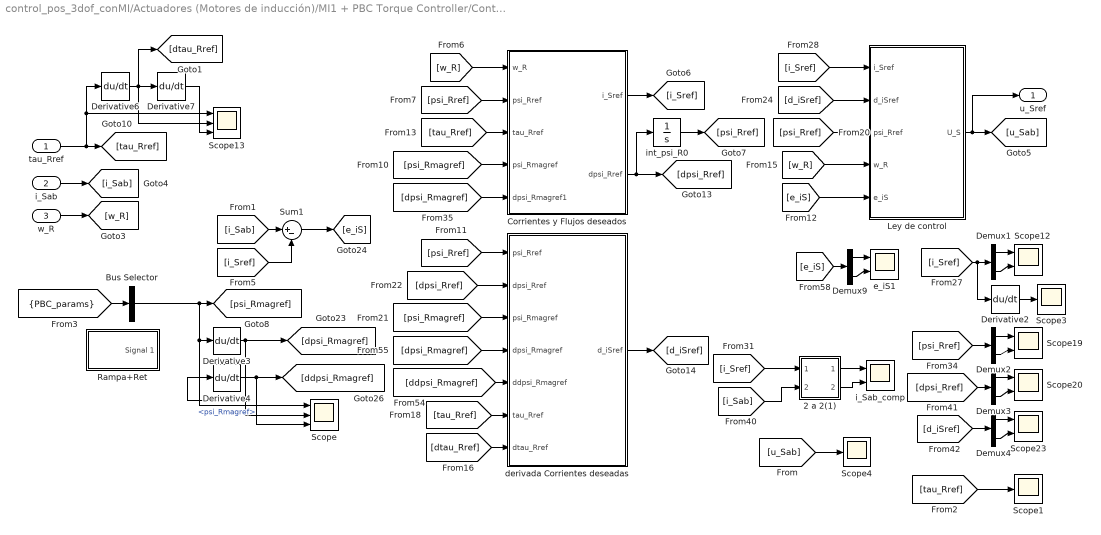
== system control_pos_3dof_conMI/Actuadores (Motores de inducción)/MI1 + PBC Torque Controller/Controlador PBC ==
  tau_Rref : Inport
  i_Sab : Inport  Port=2
  w_R : Inport  Port=3
  2 a 2(1) : Subsystem
  Bus Selector : BusSelector  OutputSignals=psi_Rmagref
  Corrientes y Flujos deseados : Subsystem
  Demux{1..4,9} (5 alike) : Demux  Outputs=2
  Derivative{2..4,6..7} (5 alike) : Derivative
  Ley de control : Subsystem
  Rampa+Ret : Subsystem  Tag=STV Subsys  LoadFcn=sigbuilder_block('load');  StartFcn=sigbuilder_block('start');  StopFcn=sigbuilder_block('stop');  ClipboardFcn=sigbuilder_block('clipboard');  mask(Sigbuilder block){tuvar=[0:10]}
      mask help: Sigbuilder GUI
      mask init:
      | if ~strcmp(get_param(bdroot(gcbh),'SimulationStatus'),'stopped') tuvar = sigbuilder_block('maskInit'); end
      settings: CopyFcn=sigbuilder_block('copy');  DeleteFcn=sigbuilder_block('delete');  ModelCloseFcn=sigbuilder_block('modelClose');  PreSaveFcn=sigbuilder_block('preSave');  PauseFcn=sigbuilder_block('pause')  ContinueFcn=sigbuilder_block('continue')  NameChangeFcn=sigbuilder_block('namechange');  OpenFcn=sigbuilder_block('open',[280.5 86.5 550.5 399.5 ]);  CloseFcn=sigbuilder_block('close');
      mask Display: plot(0, 0, 100, 100,[2, 2, 32, 32, 2], [68, 8, 8, 68, 68],[32, 2], [38, 38], [32, 19, 2],[53, 60, 44], [32, 17, 17, 2],[16, 16, 31, 31]);txt = getActiveGroup(gcbh);text(2, 100, txt,'verticalAlignment', 'top');
  Scope : Scope  NumInputPorts=3
  Scope1 : Scope
  Scope{12,19..20,23} (4 alike) : Scope  NumInputPorts=2
  Scope13 : Scope  NumInputPorts=3
  Scope3 : Scope
  Scope4 : Scope
  Sum1 : Sum  Inputs=|+-
  derivada Corrientes deseadas : Subsystem
  e_iS1 : Scope  NumInputPorts=2
  i_Sab_comp : Scope  NumInputPorts=2
  int_psi_R0 : Integrator  InitialCondition=[0.51032;0]
  u_Sref : Outport
  wires:
  Derivative3/1 -> Scope/2, Derivative4/1, [dpsi_Rmagref]
  Derivative4/1 -> [ddpsi_Rmagref], Scope/3
  Bus Selector/1 -> Scope/1, Derivative3/1, [psi_Rmagref]  "<psi_Rmagref>"
  i_Sab/1 -> [i_Sab]
  Demux1/1 -> Scope12/1
  [d_iSref] -> Demux4/1
  Demux3/2 -> Scope20/2
  Demux2/1 -> Scope19/1
  Demux1/2 -> Scope12/2
  [dpsi_Rref] -> Demux3/1
  Demux3/1 -> Scope20/1
  Demux4/1 -> Scope23/1
  [psi_Rref] -> Demux2/1
  Demux4/2 -> Scope23/2
  Demux2/2 -> Scope19/2
  [tau_Rref] -> Corrientes y Flujos deseados/3(tau_Rref)
  [w_R] -> Corrientes y Flujos deseados/1(w_R)
  int_psi_R0/1 -> [psi_Rref]
  Corrientes y Flujos deseados/2(dpsi_Rref) -> int_psi_R0/1, [dpsi_Rref]
  [psi_Rref] -> Corrientes y Flujos deseados/2(psi_Rref)
  [psi_Rmagref] -> Corrientes y Flujos deseados/4(psi_Rmagref)
  [dpsi_Rmagref] -> Corrientes y Flujos deseados/5(dpsi_Rmagref1)
  [psi_Rref] -> derivada Corrientes deseadas/1(psi_Rref)
  [dpsi_Rref] -> derivada Corrientes deseadas/2(dpsi_Rref)
  [psi_Rmagref] -> derivada Corrientes deseadas/3(psi_Rmagref)
  [dpsi_Rmagref] -> derivada Corrientes deseadas/4(dpsi_Rmagref)
  [ddpsi_Rmagref] -> derivada Corrientes deseadas/5(ddpsi_Rmagref)
  [tau_Rref] -> derivada Corrientes deseadas/6(tau_Rref)
  [dtau_Rref] -> derivada Corrientes deseadas/7(dtau_Rref)
  derivada Corrientes deseadas/1(d_iSref) -> [d_iSref]
  [e_iS] -> Demux9/1
  Demux9/1 -> e_iS1/1
  Demux9/2 -> e_iS1/2
  [i_Sab] -> Sum1/1
  [i_Sref] -> Sum1/2
  Sum1/1 -> [e_iS]
  [u_Sab] -> Scope4/1
  [i_Sref] -> Ley de control/1(i_Sref)
  [d_iSref] -> Ley de control/2(d_iSref)
  [psi_Rref] -> Ley de control/3(psi_Rref)
  [w_R] -> Ley de control/4(w_R)
  Ley de control/1(U_S) -> u_Sref/1, [u_Sab]
  [e_iS] -> Ley de control/5(e_iS)
  Derivative7/1 -> Scope13/3
  tau_Rref/1 -> Derivative6/1, Scope13/1, [tau_Rref]
  Derivative6/1 -> [dtau_Rref], Derivative7/1, Scope13/2
  2 a 2(1)/2(Out2) -> i_Sab_comp/2
  2 a 2(1)/1(Out1) -> i_Sab_comp/1
  [i_Sab] -> 2 a 2(1)/2(In2)
  [i_Sref] -> 2 a 2(1)/1(In1)
  [i_Sref] -> Derivative2/1, Demux1/1
  Derivative2/1 -> Scope3/1
  w_R/1 -> [w_R]
  [tau_Rref] -> Scope1/1
  [PBC_params] -> Bus Selector/1
  Corrientes y Flujos deseados/1(i_Sref) -> [i_Sref]

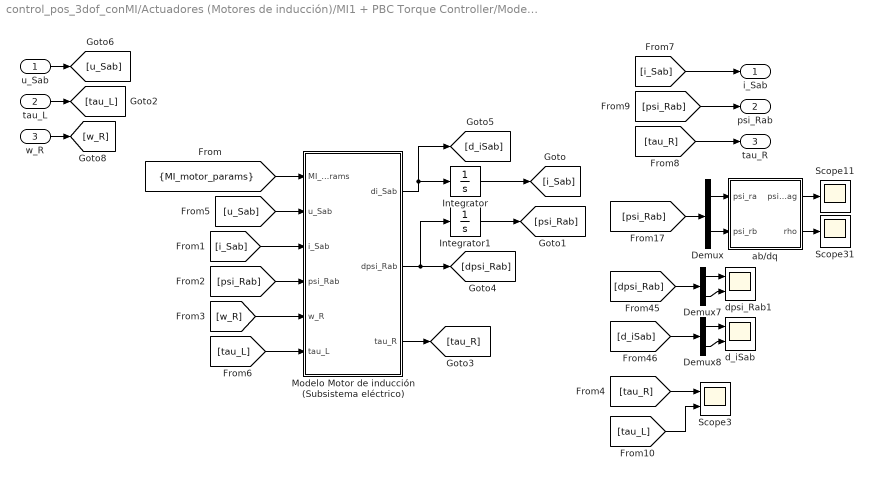
== system control_pos_3dof_conMI/Actuadores (Motores de inducción)/MI1 + PBC Torque Controller/Modelo MI (Subsistema eléctrico) ==
  u_Sab : Inport
  tau_L : Inport  Port=2
  w_R : Inport  Port=3
  Demux : Demux  Outputs=2
  Demux7 : Demux  Outputs=2
  Demux8 : Demux  Outputs=2
  Integrator : Integrator
  Integrator1 : Integrator
  Modelo Motor de inducción (Subsistema eléctrico) : MATLAB Function  TreatAsAtomicUnit=on
  Scope11 : Scope
  Scope3 : Scope  NumInputPorts=2
  Scope31 : Scope
  ab/dq : MATLAB Function  TreatAsAtomicUnit=on
  d_iSab : Scope  NumInputPorts=2
  dpsi_Rab1 : Scope  NumInputPorts=2
  i_Sab : Outport
  psi_Rab : Outport  Port=2
  tau_R : Outport  Port=3
  wires:
  Modelo Motor de inducción (Subsistema eléctrico)/1(di_Sab) -> Integrator/1, [d_iSab]
  Modelo Motor de inducción (Subsistema eléctrico)/2(dpsi_Rab) -> Integrator1/1, [dpsi_Rab]
  [w_R] -> Modelo Motor de inducción (Subsistema eléctrico)/5(w_R)
  [psi_Rab] -> Modelo Motor de inducción (Subsistema eléctrico)/4(psi_Rab)
  [i_Sab] -> Modelo Motor de inducción (Subsistema eléctrico)/3(i_Sab)
  Integrator1/1 -> [psi_Rab]
  u_Sab/1 -> [u_Sab]
  Modelo Motor de inducción (Subsistema eléctrico)/3(tau_R) -> [tau_R]
  [tau_R] -> Scope3/1
  ab/dq/1(psi_Rmag) -> Scope11/1
  [psi_Rab] -> Demux/1
  Demux7/1 -> dpsi_Rab1/1
  Demux7/2 -> dpsi_Rab1/2
  [d_iSab] -> Demux8/1
  ab/dq/2(rho) -> Scope31/1
  Demux/1 -> ab/dq/1(psi_ra)
  Demux8/2 -> d_iSab/2
  Demux8/1 -> d_iSab/1
  [dpsi_Rab] -> Demux7/1
  Demux/2 -> ab/dq/2(psi_rb)
  Integrator/1 -> [i_Sab]
  [MI_motor_params] -> Modelo Motor de inducción (Subsistema eléctrico)/1(MI_motor_params)
  [u_Sab] -> Modelo Motor de inducción (Subsistema eléctrico)/2(u_Sab)
  tau_L/1 -> [tau_L]
  [tau_L] -> Modelo Motor de inducción (Subsistema eléctrico)/6(tau_L)
  w_R/1 -> [w_R]
  [tau_R] -> tau_R/1
  [psi_Rab] -> psi_Rab/1
  [i_Sab] -> i_Sab/1
  [tau_L] -> Scope3/2

== system control_pos_3dof_conMI/Actuadores (Motores de inducción)/MI2 + PBC Torque Controller/Calculo de Potencia eléctrica ==
  u_Sab : Inport
  i_Sab : Inport  Port=2
  Blondel-Park-i_Sab : MATLAB Function  TreatAsAtomicUnit=on
  Blondel-Park-u_Sab : MATLAB Function  TreatAsAtomicUnit=on
  Demux1 : Demux  Outputs=2
  Demux2 : Demux  Outputs=2
  Demux4 : Demux  Outputs=3
  Mux : Mux  Inputs=3
  Mux1 : Mux  Inputs=3
  Product1 : Product
  Sum1 : Sum  Inputs=|+++
  P_elect : Outport
  u_S3abc : Outport  Port=2
  i_S3abc : Outport  Port=3
  wires:
  Blondel-Park-u_Sab/2(U2) -> Mux1/2
  Blondel-Park-i_Sab/2(U2) -> Mux/2
  Blondel-Park-i_Sab/1(U1) -> Mux/1
  Blondel-Park-u_Sab/3(U3) -> Mux1/3
  Blondel-Park-i_Sab/3(U3) -> Mux/3
  Sum1/1 -> P_elect/1
  Demux2/2 -> Blondel-Park-u_Sab/2(BPU2)
  Demux2/1 -> Blondel-Park-u_Sab/1(BPU1)
  Demux1/2 -> Blondel-Park-i_Sab/2(BPU2)
  Demux4/1 -> Sum1/1
  [i_S3abc] -> Product1/2
  i_Sab/1 -> Demux2/1
  Blondel-Park-u_Sab/1(U1) -> Mux1/1
  Demux1/1 -> Blondel-Park-i_Sab/1(BPU1)
  Demux4/3 -> Sum1/3
  [u_S3abc] -> Product1/1
  Demux4/2 -> Sum1/2
  Product1/1 -> Demux4/1
  u_Sab/1 -> Demux1/1
  [u_S3abc] -> u_S3abc/1
  [i_S3abc] -> i_S3abc/1
  Mux/1 -> [u_S3abc]
  Mux1/1 -> [i_S3abc]
